simulink model "Demo2"  (R2018a)
settings: Solver=VariableStepAuto  StartTime=0.0  StopTime=30  RelTol=1e-3
settings Model: Creator=aparanja  LastModifiedBy=aparanja

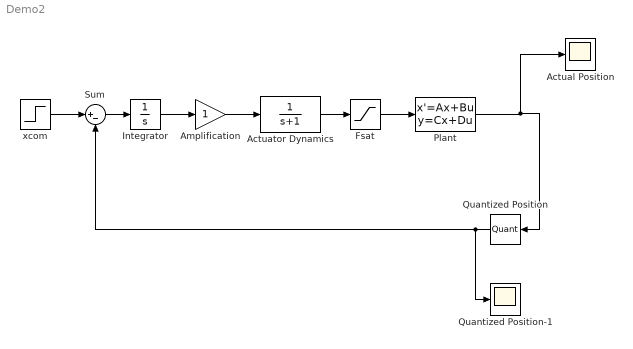
== system Demo2 ==
  Actual Position : Scope
  Actuator Dynamics : TransferFcn  Denominator=[1 1]
  Amplification : Gain
  Fsat : Saturate  UpperLimit=10  LowerLimit=-10
  Integrator : Integrator
  Plant : StateSpace  A=[0, 1; -4, -2.8]  B=[0; 1]  C=[1, 0]  D=0  InitialCondition=0
  Quantized Position : Quantizer  QuantizationInterval=0.005
  Quantized Position-1 : Scope
  Sum : Sum  Inputs=|+-
  xcom : Step  After=2  SampleTime=0
  wires:
  Plant/1 -> Quantized Position/1, Actual Position/1
  Actuator Dynamics/1 -> Fsat/1
  Fsat/1 -> Plant/1
  Quantized Position/1 -> Sum/2, Quantized Position-1/1
  xcom/1 -> Sum/1
  Sum/1 -> Integrator/1
  Amplification/1 -> Actuator Dynamics/1
  Integrator/1 -> Amplification/1
